simulink model "P4p2_integral"  (Simulink 8.3)
settings: Solver=ode1  StartTime=0.0  StopTime=inf  FixedStep=0.002  RelTol=1e-3
PostLoadFcn:
  | qc_set_target_type(getConfigSet(bdroot, 'QUARC Default Target Configuration'));
values from neighbouring files (symbols this model uses):
  A_obs = [0 1 0 0 0 0 ... (first row only)    [P4p2_init.m]    (also in P4p2_integral_init.m; P4p3_init.m)
  B_obs = [0 0 ... (first row only)    [P4p2_init.m]    (also in P4p2_integral_init.m; P4p3_init.m)
  C_obs = [1 0 0 0 0 0 ... (first row only)    [P4p2_init.m]    (also in P4p2_integral_init.m; P4p3_init.m)
  Joystick_gain_x = 1    [P4p2_init.m]    (also in P4p2_integral_init.m; P4p3_init.m)
  Joystick_gain_y = -1    [P4p2_init.m]    (also in P4p2_integral_init.m; P4p3_init.m)
  K_aug = lqr(A_aug, B_aug, Q_aug, R)    [P4p2_integral_init.m]    (also in P4p3_init.m)
  L = place(A_obs', C_obs', Pol')'    [P4p2_init.m]    (also in P4p2_integral_init.m; P4p3_init.m = place(A_obs', C_obs_not_p', Pol')')
  P = inv(C*inv(B*K-A)*B)    [P4p2_init.m]    (also in P4p2_integral_init.m; P4p3_init.m)
  v_s_star = 6.95    [P4p2_init.m]    (also in P4p2_integral_init.m; P4p3_init.m)
undefined symbols (not defined in the file or in its folder): HIL, qc_get_step_size
libraries: simulink_extras x18, quarc_library x4
settings Model: Creator=Rchan  LastModifiedBy=marmad  SimulationMode=external  ExtModeTrigDuration=5000
settings SolverCC: PositivePriorityOrder=on
settings OptimizationCC: ExpressionDepthLimit=2147483647  InitFltsAndDblsToZero=on
settings DebuggingCC: SaveWithParameterizedLinksMsg=none  MultiTaskDSMMsg=warning  MultiTaskCondExecSysMsg=none  FcnCallInpInsideContextMsg=UseLocalSettings
settings RTWCC: SystemTargetFile=quarc_win64.tlc  TemplateMakefile=quarc_default_tmf  Description=QUARC Win64 Target  ProcessScript=quarc_win64_make_rtw_hook
settings STFCustomTargetCC: TargetPreCompLibLocation=C:\PROGRA~3\QUARC\lib\2014a\win64\release  ConcurrentExecutionCompliant=on  GeneratePreprocessorConditionals=Disable all  CPPClassGenCompliant=on  SystemTargetFile=quarc_win64.tlc
settings GRTTargetCC: TargetPreCompLibLocation=C:\PROGRA~3\QUARC\lib\2014a\win64\release  ParMdlRefBuildCompliant=off  CompOptLevelCompliant=off  MatFileLogging=off  ExtMode=on  ExtModeMexFile=quarc_comm

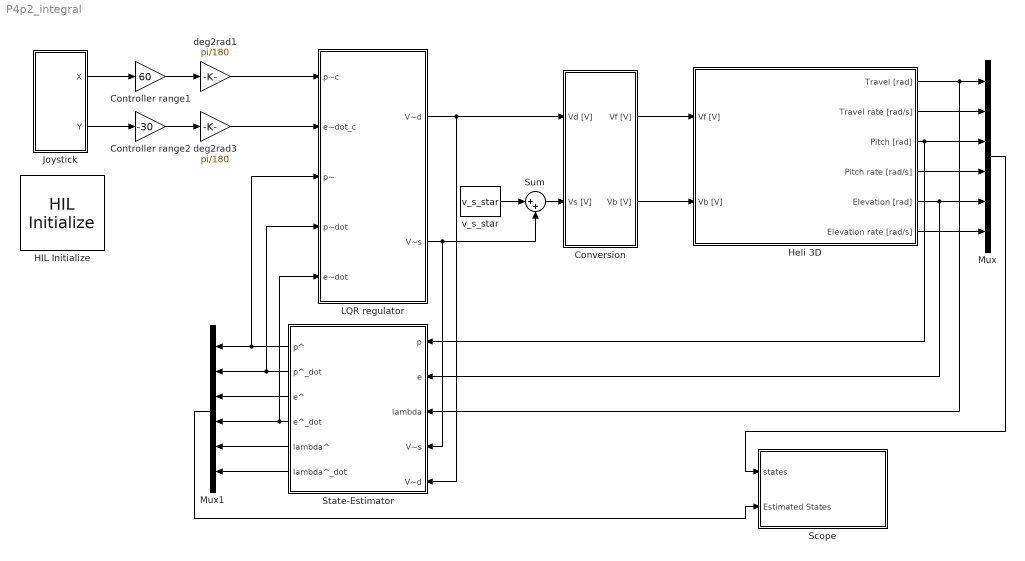
== system P4p2_integral ==
  Controller range1 : Gain  Gain=60
  Controller range2 : Gain  Gain=-30
  Conversion : Subsystem
  HIL Initialize : quarc_library/Data Acquisition/Generic/Configuration/HIL Initialize  Priority=-99  object_name=HIL-1  board_type=q8_usb  board_number=0  board_options=update_rate=normal;decimation=1  exclusive=off  active=off  hardware_clocks=[0:2]  clock_modes=[]  initial_clock_frequencies=[]  set_clock_params_at_start=off  set_clock_params_at_switch_in=off  set_clock_frequencies_at_start=off  set_clock_frequencies_at_switch_in=off  analog_input_channels=[0:7]  analog_input_maximums=10  analog_input_minimums=-10  set_analog_input_params_at_start=on  set_analog_input_params_at_switch_in=off  analog_output_channels=[0:7]  analog_output_maximums=10  analog_output_minimums=-10  initial_analog_outputs=[0]  final_analog_outputs=[0]  watchdog_analog_outputs=0  set_analog_output_params_at_start=on  set_analog_output_params_at_switch_in=off  set_analog_outputs_at_start=on  set_analog_outputs_at_switch_in=off  set_analog_outputs_at_terminate=on  set_analog_outputs_at_switch_out=off  set_analog_outputs_on_watchdog=off  digital_input_channels=[]  digital_output_channels=[]  digital_output_configuration=[]  initial_digital_outputs=[1]  final_digital_outputs=[1]  watchdog_digital_outputs=[1]  set_digital_output_params_at_start=off  set_digital_output_params_at_switch_in=off  set_digital_outputs_at_start=on  set_digital_outputs_at_switch_in=off  set_digital_outputs_at_terminate=on  set_digital_outputs_at_switch_out=off  set_digital_outputs_on_watchdog=off  encoder_channels=[0:7]  quadrature=[4]  encoder_filter_frequency=[]  initial_encoder_counts=[0]  set_encoder_params_at_start=on  set_encoder_params_at_switch_in=off  set_encoder_counts_at_start=on  set_encoder_counts_at_switch_in=off  pwm_channels=[0:7]  pwm_modes=0  pwm_frequency=99.532799999999995e6/4095  pwm_configuration=[0]  pwm_alignment=[0]  pwm_polarity=[1]  pwm_leading_deadband=[0]  pwm_trailing_deadband=[0]  initial_pwm_outputs=[0]  final_pwm_outputs=[0]  watchdog_pwm_outputs=[0]  set_pwm_params_at_start=on  set_pwm_params_at_switch_in=off  set_pwm_outputs_at_start=on  set_pwm_outputs_at_switch_in=off  set_pwm_outputs_at_terminate=on  set_pwm_outputs_at_switch_out=off  set_pwm_outputs_on_watchdog=off  other_output_channels=[]  initial_other_outputs=[]  final_other_outputs=[]  watchdog_other_outputs=[]  set_other_outputs_at_start=off  set_other_outputs_at_switch_in=off  set_other_outputs_at_terminate=off  set_other_outputs_at_switch_out=off  set_other_outputs_on_watchdog=off
  Heli 3D : Subsystem
  Joystick : Subsystem
  LQR regulator : Subsystem
  Mux : Mux  Inputs=6
  Mux1 : Mux  Inputs=6
  "Scope  " : Subsystem
  State-Estimator : Subsystem
  Sum : Sum  Inputs=|++
  deg2rad1 : Gain  Gain=pi/180
  deg2rad3 : Gain  Gain=pi/180
  v_s_star : Constant  Value=v_s_star
  wires:
  Conversion/2(Vb [V]) -> Heli 3D/2(Vb [V])
  Conversion/1(Vf [V]) -> Heli 3D/1(Vf [V])
  Sum/1 -> Conversion/2(Vs [V])
  v_s_star/1 -> Sum/1
  LQR regulator/2(V~s) -> Sum/2, State-Estimator/4("V~s ")
  Joystick/1(X) -> Controller range1/1
  Controller range1/1 -> deg2rad1/1
  deg2rad1/1 -> LQR regulator/1(p~c)
  Joystick/2(Y) -> Controller range2/1
  LQR regulator/1(V~d) -> Conversion/1(Vd [V]), State-Estimator/5(V~d)
  Heli 3D/3(Pitch [rad]) -> Mux/3, State-Estimator/1("p ")
  Controller range2/1 -> deg2rad3/1
  deg2rad3/1 -> LQR regulator/2(e~dot_c)
  Heli 3D/1(Travel [rad]) -> Mux/1, State-Estimator/3(lambda)
  State-Estimator/2(p^_dot) -> Mux1/2, LQR regulator/4(p~dot)
  State-Estimator/4(e^_dot) -> Mux1/4, LQR regulator/5(e~dot)
  State-Estimator/1("p^ ") -> Mux1/1, LQR regulator/3(p~)
  Heli 3D/5(Elevation [rad]) -> Mux/5, State-Estimator/2(e)
  Heli 3D/6(Elevation rate [rad/s]) -> Mux/6
  Heli 3D/2(Travel rate [rad/s]) -> Mux/2
  Heli 3D/4(Pitch rate [rad/s]) -> Mux/4
  State-Estimator/3(e^) -> Mux1/3
  State-Estimator/5(lambda^) -> Mux1/5
  State-Estimator/6(lambda^_dot) -> Mux1/6
  Mux/1 -> "Scope  "/1(states)
  Mux1/1 -> "Scope  "/2("Estimated States ")

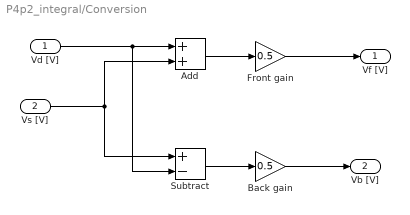
== system P4p2_integral/Conversion ==
  Vd [V] : Inport
  Vs [V] : Inport  Port=2
  Add : Sum
  Back gain : Gain  Gain=0.5
  Front gain : Gain  Gain=0.5
  Subtract : Sum  Inputs=+-
  Vf [V] : Outport
  Vb [V] : Outport  Port=2
  wires:
  Vd [V]/1 -> Subtract/2, Add/1
  Vs [V]/1 -> Subtract/1, Add/2
  Subtract/1 -> Back gain/1
  Back gain/1 -> Vb [V]/1
  Add/1 -> Front gain/1
  Front gain/1 -> Vf [V]/1

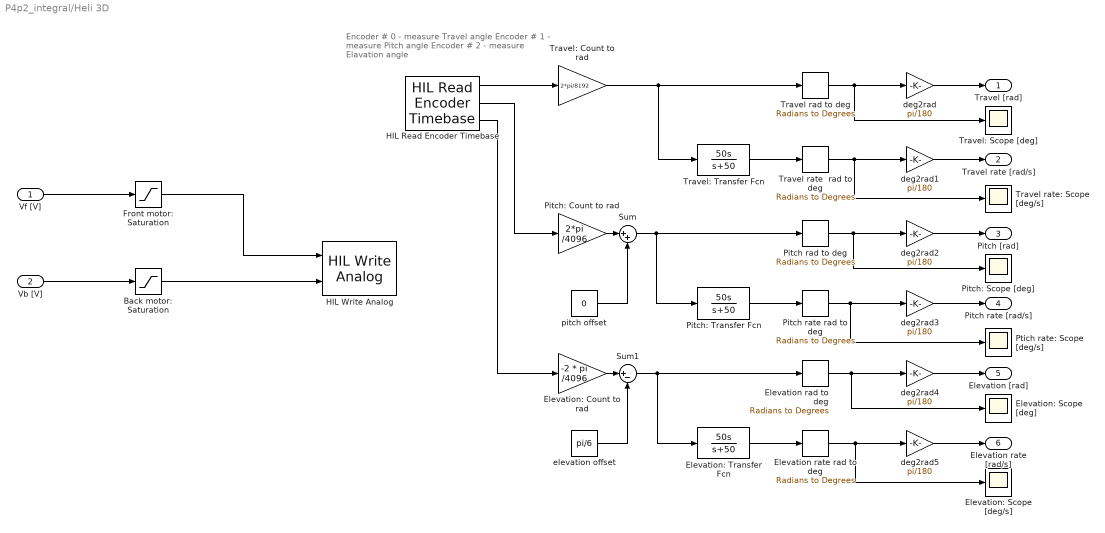
== system P4p2_integral/Heli 3D ==
  note: Encoder # 0 - measure Travel angle
      | Encoder # 1 - measure Pitch angle
      | Encoder # 2 - measure Elavation angle
  Vf [V] : Inport
  Vb [V] : Inport  Port=2
  Back motor: Saturation : Saturate  UpperLimit=5  LowerLimit=-5
  Elevation rad to deg : simulink_extras/Transformations/Radians to Degrees
  Elevation rate rad to deg : simulink_extras/Transformations/Radians to Degrees
  Elevation: Count to rad : Gain  Gain=-2 * pi /4096
  Elevation: Scope [deg/s] : Scope
      settings: YMin=-15  YMax=15  SaveName=ScopeData13
  Elevation: Scope [deg] : Scope
      settings: YMin=-32.5  YMax=0  SaveName=ScopeData12
  Elevation: Transfer Fcn : TransferFcn  Numerator=[50 0]  Denominator=[1 50]
  Front motor: Saturation : Saturate  UpperLimit=5  LowerLimit=-5
  HIL Read Encoder Timebase : quarc_library/Data Acquisition/Generic/Timebases/HIL Read Encoder Timebase  object_name=HIL-1  clock=0  channels=[0:2]  samples_in_buffer=max(ceil(1/qc_get_step_size), 1)  active=on  vector_output=off  data_type_mode=Inherit via back propagation  data_type=double
  HIL Write Analog : quarc_library/Data Acquisition/Generic/Immediate I//O/HIL Write Analog  object_name=HIL-1  channels=[0:1]  sample_time=-1  active=off  vector_input=off
  Pitch rad to deg : simulink_extras/Transformations/Radians to Degrees
  Pitch rate rad to deg : simulink_extras/Transformations/Radians to Degrees
  Pitch: Count to rad : Gain  Gain=2*pi /4096
  Pitch: Scope [deg] : Scope
      settings: YMin=-100  YMax=100  SaveName=ScopeData10
  Pitch: Transfer Fcn : TransferFcn  Numerator=[50 0]  Denominator=[1 50]
  Ptich rate: Scope [deg/s] : Scope
      settings: YMin=-15  YMax=15  SaveName=ScopeData11
  Sum : Sum  Inputs=|++
  Sum1 : Sum  Inputs=|+-
  Travel rad to deg : simulink_extras/Transformations/Radians to Degrees
  Travel rate  rad to deg : simulink_extras/Transformations/Radians to Degrees
  Travel rate: Scope [deg/s] : Scope
      settings: YMin=-15  YMax=15  SaveName=ScopeData9
  Travel: Count to rad : Gain  Gain=2*pi/8192
  Travel: Scope [deg] : Scope
      settings: YMin=-15  YMax=15  SaveName=ScopeData8
  Travel: Transfer Fcn : TransferFcn  Numerator=[50 0]  Denominator=[1 50]
  deg2rad{,1..5} (6 alike) : Gain  Gain=pi/180
  elevation offset : Constant  Value=pi/6
  pitch offset : Constant  Value=0
  Travel [rad] : Outport
  Travel rate [rad/s] : Outport  Port=2
  Pitch [rad] : Outport  Port=3
  Pitch rate [rad/s] : Outport  Port=4
  Elevation [rad] : Outport  Port=5
  Elevation rate [rad/s] : Outport  Port=6
  wires:
  HIL Read Encoder Timebase/1 -> Travel: Count to rad/1
  HIL Read Encoder Timebase/2 -> Pitch: Count to rad/1
  HIL Read Encoder Timebase/3 -> Elevation: Count to rad/1
  Travel: Count to rad/1 -> Travel: Transfer Fcn/1, Travel rad to deg/1
  Travel: Transfer Fcn/1 -> Travel rate  rad to deg/1
  Sum/1 -> Pitch: Transfer Fcn/1, Pitch rad to deg/1
  Pitch: Transfer Fcn/1 -> Pitch rate rad to deg/1
  Sum1/1 -> Elevation rad to deg/1, Elevation: Transfer Fcn/1
  Elevation: Transfer Fcn/1 -> Elevation rate rad to deg/1
  Travel rad to deg/1 -> Travel: Scope [deg]/1, deg2rad/1
  Travel rate  rad to deg/1 -> deg2rad1/1, Travel rate: Scope [deg/s]/1
  Pitch rad to deg/1 -> deg2rad2/1, Pitch: Scope [deg]/1
  Pitch rate rad to deg/1 -> deg2rad3/1, Ptich rate: Scope [deg/s]/1
  Elevation rad to deg/1 -> deg2rad4/1, Elevation: Scope [deg]/1
  Elevation rate rad to deg/1 -> deg2rad5/1, Elevation: Scope [deg/s]/1
  Vf [V]/1 -> Front motor: Saturation/1
  Vb [V]/1 -> Back motor: Saturation/1
  Front motor: Saturation/1 -> HIL Write Analog/1
  Back motor: Saturation/1 -> HIL Write Analog/2
  deg2rad/1 -> Travel [rad]/1
  deg2rad1/1 -> Travel rate [rad/s]/1
  deg2rad2/1 -> Pitch [rad]/1
  deg2rad3/1 -> Pitch rate [rad/s]/1
  deg2rad4/1 -> Elevation [rad]/1
  deg2rad5/1 -> Elevation rate [rad/s]/1
  Pitch: Count to rad/1 -> Sum/1
  pitch offset/1 -> Sum/2
  Elevation: Count to rad/1 -> Sum1/1
  elevation offset/1 -> Sum1/2

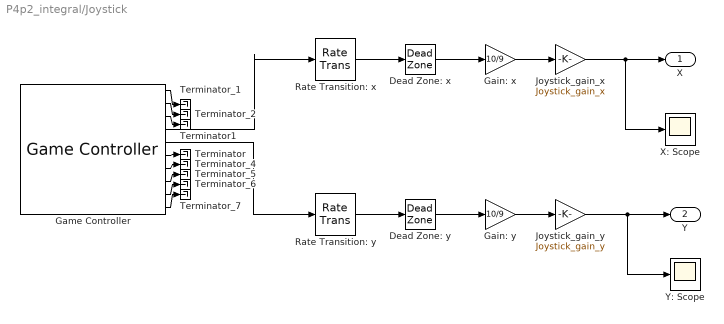
== system P4p2_integral/Joystick ==
  Dead Zone: x : DeadZone  LowerValue=-0.1  UpperValue=0.1  SaturateOnIntegerOverflow=on
  Dead Zone: y : DeadZone  LowerValue=-0.1  UpperValue=0.1  SaturateOnIntegerOverflow=on
  Gain: x : Gain  Gain=10/9
  Gain: y : Gain  Gain=10/9
  Game Controller : quarc_library/Devices/Peripherals/Target/Game Controller  controller=1  buffer_size=12  deadzone=[]  saturation=[]  sample_time=max(qc_get_step_size, 0.01)  auto_center=off  enabled=on
  Joystick_gain_x : Gain  Gain=Joystick_gain_x
  Joystick_gain_y : Gain  Gain=Joystick_gain_y
  Rate Transition: x : RateTransition
  Rate Transition: y : RateTransition
  Terminator : Terminator
  Terminator1 : Terminator
  Terminator_{1..2,4..7} (6 alike) : Terminator
  X: Scope : Scope
      settings: YMin=-1  YMax=1  SaveName=ScopeData7
  Y: Scope : Scope
      settings: YMin=-10  YMax=10  SaveName=ScopeData5
  X : Outport
  Y : Outport  Port=2
  wires:
  Rate Transition: y/1 -> Dead Zone: y/1
  Rate Transition: x/1 -> Dead Zone: x/1
  Game Controller/5 -> Rate Transition: y/1
  Game Controller/4 -> Rate Transition: x/1
  Game Controller/1 -> Terminator_1/1
  Game Controller/2 -> Terminator_2/1
  Game Controller/7 -> Terminator_4/1
  Game Controller/8 -> Terminator_5/1
  Game Controller/9 -> Terminator_6/1
  Game Controller/10 -> Terminator_7/1
  Game Controller/3 -> Terminator1/1
  Game Controller/6 -> Terminator/1
  Dead Zone: x/1 -> Gain: x/1
  Dead Zone: y/1 -> Gain: y/1
  Gain: x/1 -> Joystick_gain_x/1
  Gain: y/1 -> Joystick_gain_y/1
  Joystick_gain_x/1 -> X/1, X: Scope/1
  Joystick_gain_y/1 -> Y: Scope/1, Y/1

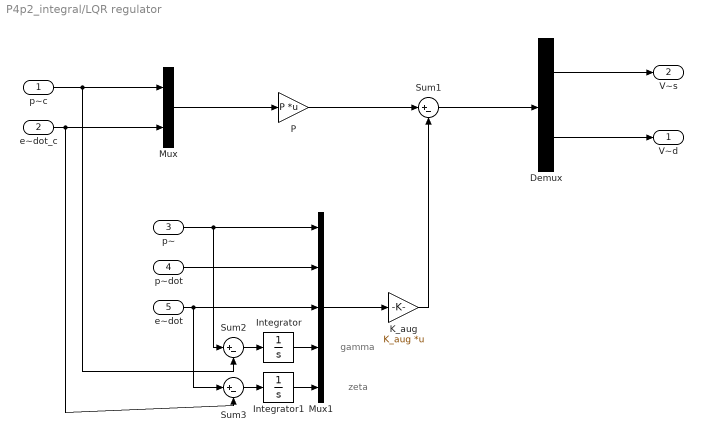
== system P4p2_integral/LQR regulator ==
  note: zeta
  note: gamma
  p~c : Inport
  e~dot_c : Inport  Port=2
  p~ : Inport  Port=3
  p~dot : Inport  Port=4
  e~dot : Inport  Port=5
  Demux : Demux  Outputs=2
  Integrator : Integrator
  Integrator1 : Integrator
  "K_aug " : Gain  Gain=K_aug  Multiplication=Matrix(K*u)
  Mux : Mux  Inputs=2
  Mux1 : Mux  Inputs=5
  P : Gain  Gain=P  Multiplication=Matrix(K*u)
  Sum1 : Sum  Inputs=|+-
  Sum2 : Sum  Inputs=|+-
  Sum3 : Sum  Inputs=|+-
  V~d : Outport
  V~s : Outport  Port=2
  wires:
  p~c/1 -> Mux/1, Sum2/2
  e~dot_c/1 -> Sum3/2, Mux/2
  "K_aug "/1 -> Sum1/2
  p~dot/1 -> Mux1/2
  p~/1 -> Mux1/1, Sum2/1
  Mux/1 -> P/1
  P/1 -> Sum1/1
  e~dot/1 -> Mux1/3, Sum3/1
  Mux1/1 -> "K_aug "/1
  Sum1/1 -> Demux/1
  Demux/1 -> V~s/1
  Demux/2 -> V~d/1
  Sum2/1 -> Integrator/1
  Sum3/1 -> Integrator1/1
  Integrator/1 -> Mux1/4
  Integrator1/1 -> Mux1/5

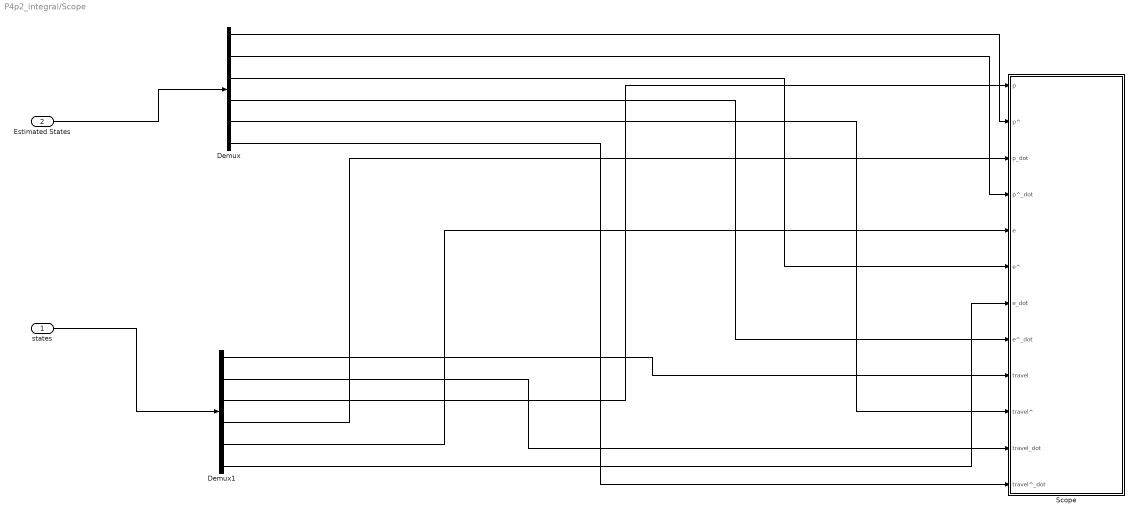
== system P4p2_integral/Scope   ==
  states : Inport
  "Estimated States " : Inport  Port=2
  Demux : Demux  Outputs=6
  Demux1 : Demux  Outputs=6
  Scope : Subsystem
  wires:
  Demux1/4 -> Scope/3(p_dot)
  Demux1/3 -> Scope/1(p)
  Demux1/2 -> Scope/11(travel_dot)
  Demux/2 -> Scope/4(p^_dot)
  Demux/1 -> Scope/2(p^)
  Demux1/1 -> Scope/9(travel)
  "Estimated States "/1 -> Demux/1
  Demux/4 -> Scope/8(e^_dot)
  Demux/5 -> Scope/10(travel^)
  Demux1/6 -> Scope/7(e_dot)
  Demux/3 -> Scope/6(e^)
  states/1 -> Demux1/1
  Demux/6 -> Scope/12(travel^_dot)
  Demux1/5 -> Scope/5(e)

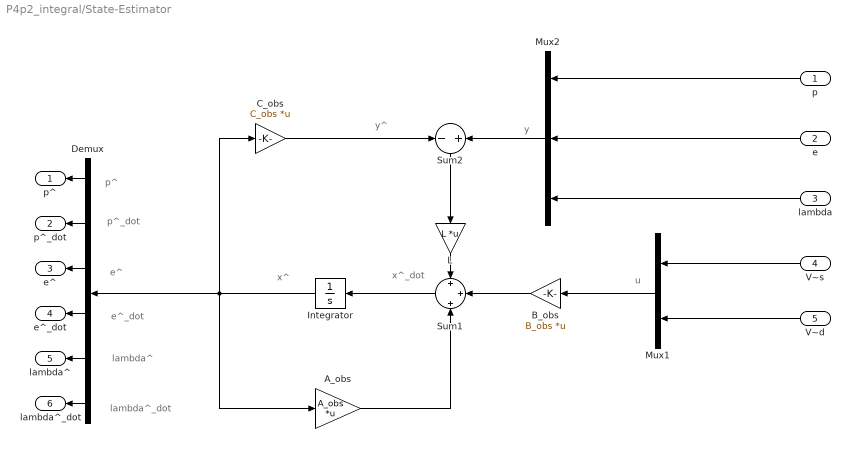
== system P4p2_integral/State-Estimator ==
  note: y^
  note: x^
  note: x^_dot
  note: y
  note: u
  note: lambda^_dot
  note: lambda^
  note: e^_dot
  note: e^
  note: p^_dot
  note: p^
  "p " : Inport
  e : Inport  Port=2
  lambda : Inport  Port=3
  "V~s " : Inport  Port=4
  V~d : Inport  Port=5
  A_obs : Gain  Gain=A_obs  Multiplication=Matrix(K*u)
  "B_obs " : Gain  Gain=B_obs  Multiplication=Matrix(K*u)
  C_obs : Gain  Gain=C_obs  Multiplication=Matrix(K*u)
  Demux : Demux  Outputs=6
  Integrator : Integrator
  L : Gain  Gain=L  Multiplication=Matrix(K*u)
  Mux1 : Mux  Inputs=2
  Mux2 : Mux  Inputs=3
  Sum1 : Sum  Inputs=+|+|+
  Sum2 : Sum  Inputs=-|+
  "p^ " : Outport
  p^_dot : Outport  Port=2
  e^ : Outport  Port=3
  e^_dot : Outport  Port=4
  lambda^ : Outport  Port=5
  lambda^_dot : Outport  Port=6
  wires:
  Sum2/1 -> L/1
  Sum1/1 -> Integrator/1
  e/1 -> Mux2/2
  Mux2/1 -> Sum2/2
  L/1 -> Sum1/1
  A_obs/1 -> Sum1/3
  lambda/1 -> Mux2/3
  Integrator/1 -> C_obs/1, Demux/1, A_obs/1
  C_obs/1 -> Sum2/1
  Demux/5 -> lambda^/1
  Demux/1 -> "p^ "/1
  Demux/4 -> e^_dot/1
  Demux/3 -> e^/1
  "p "/1 -> Mux2/1
  Demux/6 -> lambda^_dot/1
  Demux/2 -> p^_dot/1
  V~d/1 -> Mux1/2
  Mux1/1 -> "B_obs "/1
  "B_obs "/1 -> Sum1/2
  "V~s "/1 -> Mux1/1

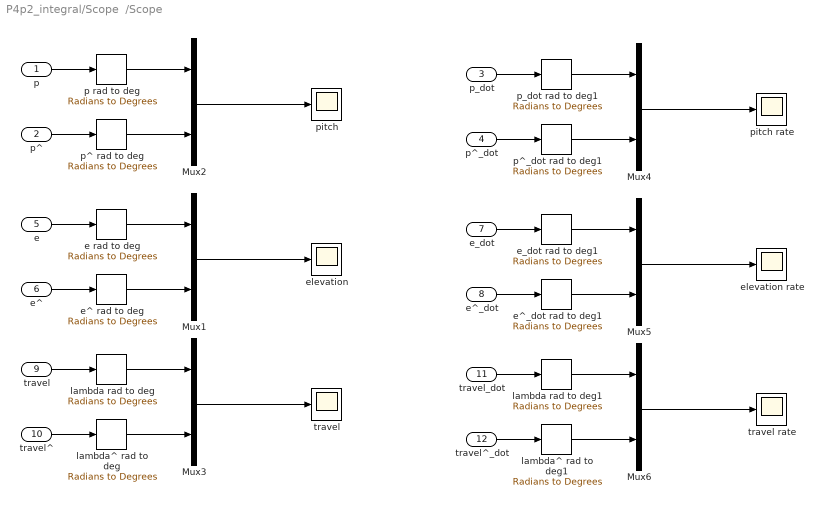
== system P4p2_integral/Scope  /Scope ==
  p : Inport
  p^ : Inport  Port=2
  p_dot : Inport  Port=3
  p^_dot : Inport  Port=4
  e : Inport  Port=5
  e^ : Inport  Port=6
  e_dot : Inport  Port=7
  e^_dot : Inport  Port=8
  travel : Inport  Port=9
  travel^ : Inport  Port=10
  travel_dot : Inport  Port=11
  travel^_dot : Inport  Port=12
  Mux{1..6} (6 alike) : Mux  Inputs=2
  e rad to deg : simulink_extras/Transformations/Radians to Degrees
  e^ rad to deg : simulink_extras/Transformations/Radians to Degrees
  e^_dot rad to deg1 : simulink_extras/Transformations/Radians to Degrees
  e_dot rad to deg1 : simulink_extras/Transformations/Radians to Degrees
  elevation : Scope
      settings: YMin=-30  YMax=30  SaveName=ScopeData4
  elevation rate : Scope
      settings: SaveName=ScopeData16
  lambda rad to deg : simulink_extras/Transformations/Radians to Degrees
  lambda rad to deg1 : simulink_extras/Transformations/Radians to Degrees
  lambda^ rad to deg : simulink_extras/Transformations/Radians to Degrees
  lambda^ rad to deg1 : simulink_extras/Transformations/Radians to Degrees
  p rad to deg : simulink_extras/Transformations/Radians to Degrees
  p^ rad to deg : simulink_extras/Transformations/Radians to Degrees
  p^_dot rad to deg1 : simulink_extras/Transformations/Radians to Degrees
  p_dot rad to deg1 : simulink_extras/Transformations/Radians to Degrees
  pitch : Scope
      settings: YMin=-65  YMax=65  SaveName=ScopeData14
  pitch rate : Scope
      settings: SaveName=ScopeData15
  "travel " : Scope
      settings: YMin=4825  YMax=5200  SaveName=ScopeData6
  travel rate : Scope
      settings: YMin=-90  YMax=90  SaveName=ScopeData17
  wires:
  travel/1 -> lambda rad to deg/1
  p^ rad to deg/1 -> Mux2/2
  e^/1 -> e^ rad to deg/1
  p rad to deg/1 -> Mux2/1
  p/1 -> p rad to deg/1
  Mux3/1 -> "travel "/1
  Mux1/1 -> elevation/1
  e/1 -> e rad to deg/1
  p^/1 -> p^ rad to deg/1
  lambda rad to deg/1 -> Mux3/1
  e^ rad to deg/1 -> Mux1/2
  e rad to deg/1 -> Mux1/1
  lambda^ rad to deg/1 -> Mux3/2
  travel^/1 -> lambda^ rad to deg/1
  Mux2/1 -> pitch/1
  p^_dot rad to deg1/1 -> Mux4/2
  p_dot rad to deg1/1 -> Mux4/1
  p_dot/1 -> p_dot rad to deg1/1
  p^_dot/1 -> p^_dot rad to deg1/1
  Mux4/1 -> pitch rate/1
  e^_dot/1 -> e^_dot rad to deg1/1
  Mux5/1 -> elevation rate/1
  e_dot/1 -> e_dot rad to deg1/1
  e^_dot rad to deg1/1 -> Mux5/2
  e_dot rad to deg1/1 -> Mux5/1
  travel_dot/1 -> lambda rad to deg1/1
  Mux6/1 -> travel rate/1
  lambda rad to deg1/1 -> Mux6/1
  lambda^ rad to deg1/1 -> Mux6/2
  travel^_dot/1 -> lambda^ rad to deg1/1
